simulink model "updated_target_driver_2026_withVariants_MPC"  (R2024b)
settings: Solver=FixedStepDiscrete  StartTime=0.0  StopTime=running_time  FixedStep=dt_s  RelTol=1e-3
values from neighbouring files (symbols this model uses):
  A = gamma_2*gamma_3*Thrust_desired    [force2voltage.m]
  a2_lb = -0.25    [target_driver_setup_2022_Ctrl_V_2_4.m]    (also in target_driver_setup_2022_Ctrl_V_2_4_geometric.m; target_driver_setup_mpc_12msdelay.m; target_driver_setup_mpc_andWLQP.m)
  a2_openloop = -0    (= 0)    [target_driver_setup_2022_Ctrl_V_2_4.m]    (also in target_driver_setup_2022_Ctrl_V_2_4_geometric.m; target_driver_setup_mpc_12msdelay.m; target_driver_setup_mpc_andWLQP.m)
  a2_ub = 0.25    [target_driver_setup_2022_Ctrl_V_2_4.m]    (also in target_driver_setup_2022_Ctrl_V_2_4_geometric.m; target_driver_setup_mpc_12msdelay.m; target_driver_setup_mpc_andWLQP.m)
  adaptive_flag = 0    [target_driver_setup_2022_Ctrl_V_2_4.m]    (also in target_driver_setup_2022_Ctrl_V_2_4_geometric.m; target_driver_setup_mpc_12msdelay.m = 1; target_driver_setup_mpc_andWLQP.m = 1)
  adaptive_gain = [gamma_adaptive, adaptive_roll_limit, adaptive_pitch_limit, adaptive_yaw_limit, c_2_adaptive, gamma_lateral_adaptive, adaptive_x_limit, adaptive_y_limit, adaptive_z_limit, c_1_adaptive]    [target_driver_setup_2022_Ctrl_V_2_4.m]    (also in target_driver_setup_2022_Ctrl_V_2_4_geometric.m; target_driver_setup_mpc_12msdelay.m; target_driver_setup_mpc_andWLQP.m)
  adaptive_lateral_flag = 0    [target_driver_setup_2022_Ctrl_V_2_4.m]    (also in target_driver_setup_2022_Ctrl_V_2_4_geometric.m; target_driver_setup_mpc_12msdelay.m = 1; target_driver_setup_mpc_andWLQP.m = 1)
  adaptive_pitch_init = 0    [target_driver_setup_2022_Ctrl_V_2_4.m]    (also in target_driver_setup_2022_Ctrl_V_2_4_geometric.m; target_driver_setup_mpc_12msdelay.m; target_driver_setup_mpc_andWLQP.m)
  adaptive_pitch_limit = 0.1/(scale^2)    (= 1e-07)    [target_driver_setup_2022_Ctrl_V_2_4.m]    (also in target_driver_setup_2022_Ctrl_V_2_4_geometric.m = 3e-07; target_driver_setup_mpc_12msdelay.m; target_driver_setup_mpc_andWLQP.m)
  adaptive_pitch_limit_low = -adaptive_pitch_limit    (= -1e-07)    [target_driver_setup_2022_Ctrl_V_2_4.m]    (also in target_driver_setup_2022_Ctrl_V_2_4_geometric.m = -3e-07; target_driver_setup_mpc_12msdelay.m; target_driver_setup_mpc_andWLQP.m)
  adaptive_roll_init = 0    [target_driver_setup_2022_Ctrl_V_2_4.m]    (also in target_driver_setup_2022_Ctrl_V_2_4_geometric.m; target_driver_setup_mpc_12msdelay.m; target_driver_setup_mpc_andWLQP.m)
  adaptive_roll_limit = 0.3/(scale^2)    (= 3e-07)    [target_driver_setup_2022_Ctrl_V_2_4.m]    (also in target_driver_setup_2022_Ctrl_V_2_4_geometric.m; target_driver_setup_mpc_12msdelay.m; target_driver_setup_mpc_andWLQP.m)
  adaptive_roll_limit_low = -adaptive_roll_limit    (= -3e-07)    [target_driver_setup_2022_Ctrl_V_2_4.m]    (also in target_driver_setup_2022_Ctrl_V_2_4_geometric.m; target_driver_setup_mpc_12msdelay.m; target_driver_setup_mpc_andWLQP.m)
  adaptive_x_init = 0    [target_driver_setup_2022_Ctrl_V_2_4.m]    (also in target_driver_setup_2022_Ctrl_V_2_4_geometric.m; target_driver_setup_mpc_12msdelay.m; target_driver_setup_mpc_andWLQP.m)
  adaptive_x_limit = 0.15/(scale)    (= 0.00015)    [target_driver_setup_2022_Ctrl_V_2_4.m]    (also in target_driver_setup_2022_Ctrl_V_2_4_geometric.m = 7.5e-05; target_driver_setup_mpc_12msdelay.m; target_driver_setup_mpc_andWLQP.m)
  adaptive_x_limit_low = -adaptive_x_limit    (= -0.00015)    [target_driver_setup_2022_Ctrl_V_2_4.m]    (also in target_driver_setup_2022_Ctrl_V_2_4_geometric.m = -7.5e-05; target_driver_setup_mpc_12msdelay.m; target_driver_setup_mpc_andWLQP.m)
  adaptive_y_init = 0    [target_driver_setup_2022_Ctrl_V_2_4.m]    (also in target_driver_setup_2022_Ctrl_V_2_4_geometric.m; target_driver_setup_mpc_12msdelay.m; target_driver_setup_mpc_andWLQP.m)
  adaptive_y_limit = 0.15/(scale)    (= 0.00015)    [target_driver_setup_2022_Ctrl_V_2_4.m]    (also in target_driver_setup_2022_Ctrl_V_2_4_geometric.m = 7.5e-05; target_driver_setup_mpc_12msdelay.m; target_driver_setup_mpc_andWLQP.m)
  adaptive_y_limit_low = -adaptive_y_limit    (= -0.00015)    [target_driver_setup_2022_Ctrl_V_2_4.m]    (also in target_driver_setup_2022_Ctrl_V_2_4_geometric.m = -7.5e-05; target_driver_setup_mpc_12msdelay.m; target_driver_setup_mpc_andWLQP.m)
  adaptive_yaw_init = 0    [target_driver_setup_2022_Ctrl_V_2_4.m]    (also in target_driver_setup_2022_Ctrl_V_2_4_geometric.m; target_driver_setup_mpc_12msdelay.m; target_driver_setup_mpc_andWLQP.m)
  adaptive_yaw_limit = 0.035/(scale^2)    (= 3.5e-08)    [target_driver_setup_2022_Ctrl_V_2_4.m]    (also in target_driver_setup_2022_Ctrl_V_2_4_geometric.m; target_driver_setup_mpc_12msdelay.m; target_driver_setup_mpc_andWLQP.m)
  adaptive_yaw_limit_low = -adaptive_yaw_limit    (= -3.5e-08)    [target_driver_setup_2022_Ctrl_V_2_4.m]    (also in target_driver_setup_2022_Ctrl_V_2_4_geometric.m; target_driver_setup_mpc_12msdelay.m; target_driver_setup_mpc_andWLQP.m)
  adaptive_z_init = 0/scale    (= 0)    [target_driver_setup_2022_Ctrl_V_2_4.m]    (also in target_driver_setup_2022_Ctrl_V_2_4_geometric.m; target_driver_setup_mpc_12msdelay.m; target_driver_setup_mpc_andWLQP.m)
  adaptive_z_limit = 0.20/(scale)    (= 0.0002)    [target_driver_setup_2022_Ctrl_V_2_4.m]    (also in target_driver_setup_2022_Ctrl_V_2_4_geometric.m = 0.0008; target_driver_setup_mpc_12msdelay.m = 0.0008; target_driver_setup_mpc_andWLQP.m = 0.0008)
  adaptive_z_limit_low = -adaptive_z_limit/1    (= -0.0002)    [target_driver_setup_2022_Ctrl_V_2_4.m]    (also in target_driver_setup_2022_Ctrl_V_2_4_geometric.m = -0.0008; target_driver_setup_mpc_12msdelay.m = -0.0008; target_driver_setup_mpc_andWLQP.m = -0.0008)
  att_s = 500    [target_driver_setup_2022_Ctrl_V_2_4.m]    (also in target_driver_setup_2022_Ctrl_V_2_4_geometric.m; target_driver_setup_mpc_12msdelay.m; target_driver_setup_mpc_andWLQP.m)
  b_1_d_desired = [1,0,0]    [target_driver_setup_2022_Ctrl_V_2_4.m]    (also in target_driver_setup_2022_Ctrl_V_2_4_geometric.m; target_driver_setup_mpc_12msdelay.m; target_driver_setup_mpc_andWLQP.m)
  closedloop_flag = 1    [target_driver_setup_2022_Ctrl_V_2_4.m]    (also in target_driver_setup_2022_Ctrl_V_2_4_geometric.m = 0; target_driver_setup_mpc_12msdelay.m = 0; target_driver_setup_mpc_andWLQP.m = 0)
  control_gain = [k_x,k_v, k_R, k_Omega, k_z, k_vz, k_Rx]    [target_driver_setup_2022_Ctrl_V_2_4.m]    (also in target_driver_setup_2022_Ctrl_V_2_4_geometric.m = [k_x,k_v,k_R,k_Omega_pitch,k_Omega_roll,k_z,k_vz,k_Rx]; target_driver_setup_mpc_12msdelay.m = [k_x, k_v, k_R, k_Omega, k_z, k_vz, k_Rx,                  k; target_driver_setup_mpc_andWLQP.m = [k_x, k_v, k_R, k_Omega, k_z, k_vz, k_Rx,                  k)
  delay = delay-vicon_sample_cycle/2    [target_driver_setup_2022_Ctrl_V_2_4.m]    (also in target_driver_setup_2022_Ctrl_V_2_4_geometric.m; target_driver_setup_mpc_12msdelay.m; target_driver_setup_mpc_andWLQP.m)
  drv_amp = abs((vleft_p2p-vright_p2p))/2+min(vleft_p2p,vright_p2p)    [Wing_traj_to_Voltage.m]    (also in force2voltage.m; target_driver_setup_2022_Ctrl_V_2_4.m = 300; target_driver_setup_2022_Ctrl_V_2_4_geometric.m = 133; target_driver_setup_mpc_12msdelay.m = 150)
  drv_bias = max_drv_bias    (= 300)    [target_driver_setup_2022_Ctrl_V_2_4.m]    (also in target_driver_setup_2022_Ctrl_V_2_4_geometric.m = 200; target_driver_setup_mpc_12msdelay.m = 200; target_driver_setup_mpc_andWLQP.m = 200)
  drv_pitch_left = vleft_pitch    [Wing_traj_to_Voltage.m]    (also in force2voltage.m = 0; target_driver_setup_2022_Ctrl_V_2_4.m = 0; target_driver_setup_2022_Ctrl_V_2_4_geometric.m = 0; target_driver_setup_mpc_12msdelay.m = 9.05)
  drv_pitch_right = vright_pitch    [Wing_traj_to_Voltage.m]    (also in force2voltage.m = 0; target_driver_setup_2022_Ctrl_V_2_4.m = 0; target_driver_setup_2022_Ctrl_V_2_4_geometric.m = 0; target_driver_setup_mpc_12msdelay.m = 9.05)
  drv_roll = (vleft_p2p-vright_p2p)/4    [Wing_traj_to_Voltage.m]    (also in force2voltage.m; target_driver_setup_2022_Ctrl_V_2_4.m = 0; target_driver_setup_2022_Ctrl_V_2_4_geometric.m = -0.001; target_driver_setup_mpc_12msdelay.m = -0.001)
  dt_s = 1e-3    (= 0.001)    [target_driver_setup_2022_Ctrl_V_2_4.m]    (also in target_driver_setup_2022_Ctrl_V_2_4_geometric.m = 0.0002; target_driver_setup_mpc_12msdelay.m = 0.0002; target_driver_setup_mpc_andWLQP.m = 0.0002)
  f_fin = f    (= 180)    [target_driver_setup_2022_Ctrl_V_2_4.m]    (also in target_driver_setup_2022_Ctrl_V_2_4_geometric.m = 155; target_driver_setup_mpc_12msdelay.m = 155; target_driver_setup_mpc_andWLQP.m = 155)
  f_int = f    (= 180)    [target_driver_setup_2022_Ctrl_V_2_4.m]    (also in target_driver_setup_2022_Ctrl_V_2_4_geometric.m = 155; target_driver_setup_mpc_12msdelay.m = 155; target_driver_setup_mpc_andWLQP.m = 155)
  g = 9.8    [target_driver_setup_2022_Ctrl_V_2_4.m]    (also in target_driver_setup_2022_Ctrl_V_2_4_geometric.m; target_driver_setup_mpc_12msdelay.m; target_driver_setup_mpc_andWLQP.m = 9.81; test_full_attitude_mpc.m = 9.81)
  I_moment_vec = [Ixx, Iyy, Izz]    [target_driver_setup_2022_Ctrl_V_2_4.m]    (also in target_driver_setup_2022_Ctrl_V_2_4_geometric.m; target_driver_setup_mpc_12msdelay.m; target_driver_setup_mpc_andWLQP.m)
  k_tau_vec = [k_tau_roll;k_tau_pitch]    [target_driver_setup_2022_Ctrl_V_2_4_geometric.m]    (also in target_driver_setup_mpc_12msdelay.m; target_driver_setup_mpc_andWLQP.m)
  landing_flag = 0    [target_driver_setup_2022_Ctrl_V_2_4.m]    (also in target_driver_setup_2022_Ctrl_V_2_4_geometric.m; target_driver_setup_mpc_12msdelay.m; target_driver_setup_mpc_andWLQP.m)
  landing_parameter = [start_delay+T,transition_rate, rising_time, falling_time, landing_rising_time, landing_z_decrease, landing_y_decrease, landing_x_decrease]    [target_driver_setup_2022_Ctrl_V_2_4.m]    (also in target_driver_setup_2022_Ctrl_V_2_4_geometric.m; target_driver_setup_mpc_12msdelay.m; target_driver_setup_mpc_andWLQP.m)
  low_bound = -8    [target_driver_setup_2022_Ctrl_V_2_4.m]    (also in target_driver_setup_2022_Ctrl_V_2_4_geometric.m = -5; target_driver_setup_mpc_12msdelay.m = -10; target_driver_setup_mpc_andWLQP.m = -10)
  low_bound_eR = -0.8    [target_driver_setup_2022_Ctrl_V_2_4.m]    (also in target_driver_setup_2022_Ctrl_V_2_4_geometric.m = -1.2; target_driver_setup_mpc_12msdelay.m = -1.2; target_driver_setup_mpc_andWLQP.m = -1.2)
  low_bound_vx = -0.5    [target_driver_setup_2022_Ctrl_V_2_4.m]    (also in target_driver_setup_2022_Ctrl_V_2_4_geometric.m; target_driver_setup_mpc_12msdelay.m; target_driver_setup_mpc_andWLQP.m)
  low_bound_vy = -0.5    [target_driver_setup_2022_Ctrl_V_2_4.m]    (also in target_driver_setup_2022_Ctrl_V_2_4_geometric.m; target_driver_setup_mpc_12msdelay.m; target_driver_setup_mpc_andWLQP.m)
  low_bound_vz = -0.5    [target_driver_setup_2022_Ctrl_V_2_4.m]    (also in target_driver_setup_2022_Ctrl_V_2_4_geometric.m; target_driver_setup_mpc_12msdelay.m; target_driver_setup_mpc_andWLQP.m)
  low_bound_x = -0.06    [target_driver_setup_2022_Ctrl_V_2_4.m]    (also in target_driver_setup_2022_Ctrl_V_2_4_geometric.m = -0.1; target_driver_setup_mpc_12msdelay.m = -0.6; target_driver_setup_mpc_andWLQP.m = -0.6)
  low_bound_y = -0.06    [target_driver_setup_2022_Ctrl_V_2_4.m]    (also in target_driver_setup_2022_Ctrl_V_2_4_geometric.m; target_driver_setup_mpc_12msdelay.m = -0.6; target_driver_setup_mpc_andWLQP.m = -0.6)
  low_bound_z = -0.04    [target_driver_setup_2022_Ctrl_V_2_4.m]    (also in target_driver_setup_2022_Ctrl_V_2_4_geometric.m; target_driver_setup_mpc_12msdelay.m = -0.1; target_driver_setup_mpc_andWLQP.m = -0.1)
  m = t <= t_zoom    [plot_roll_torque_cmd_vs_actual.m]    (also in plot_roll_torque_cmd_vs_actual_flightlog.m = t >= t0 & t <= t1; target_driver_setup_2022_Ctrl_V_2_4.m = 0.000124; target_driver_setup_2022_Ctrl_V_2_4_geometric.m = 8.5655e-05; target_driver_setup_mpc_12msdelay.m = 8.5655e-05)
  params_vec = [params_opt.delta_1, params_opt.delta_2, params_opt.delta_3,      params_opt.gamma_1, params_opt.gamma_2_1, params_opt.gamma_3,      params_opt.eta, params_opt.nu, params_opt.mu]'    [force2voltage_tuningSandbox.m]    (also in target_driver_setup_2022_Ctrl_V_2_4.m = [params_opt.delta_1, params_opt.delta_2, params_opt.delta_3,; target_driver_setup_2022_Ctrl_V_2_4_geometric.m = [params_opt.delta_1, params_opt.delta_2, params_opt.delta_3,; target_driver_setup_mpc_12msdelay.m = [params_opt.delta_1, params_opt.delta_2, params_opt.delta_3,; target_driver_setup_mpc_andWLQP.m = [params_opt.delta_1, params_opt.delta_2, params_opt.delta_3,)
  phase = 0    [target_driver_setup_2022_Ctrl_V_2_4.m]    (also in target_driver_setup_2022_Ctrl_V_2_4_geometric.m; target_driver_setup_mpc_12msdelay.m; target_driver_setup_mpc_andWLQP.m)
  r_desired = [default_x, default_y,z_desired]    [target_driver_setup_2022_Ctrl_V_2_4.m]    (also in target_driver_setup_2022_Ctrl_V_2_4_geometric.m; target_driver_setup_mpc_12msdelay.m; target_driver_setup_mpc_andWLQP.m)
  roll_offset_angle = 0    [target_driver_setup_2022_Ctrl_V_2_4.m]    (also in target_driver_setup_2022_Ctrl_V_2_4_geometric.m; target_driver_setup_mpc_12msdelay.m; target_driver_setup_mpc_andWLQP.m)
  running_time = start_delay+total_T    (= 9)    [target_driver_setup_2022_Ctrl_V_2_4.m]    (also in target_driver_setup_2022_Ctrl_V_2_4_geometric.m = 10; target_driver_setup_mpc_12msdelay.m = 0.5; target_driver_setup_mpc_andWLQP.m = 10)
  running_time_control = start_delay_control+total_T+0.0    (= 7.1)    [target_driver_setup_2022_Ctrl_V_2_4.m]    (also in target_driver_setup_2022_Ctrl_V_2_4_geometric.m = 10; target_driver_setup_mpc_12msdelay.m = 0.5; target_driver_setup_mpc_andWLQP.m = 10)
  sampling_f = 10000    [target_driver_setup_2022_Ctrl_V_2_4.m]    (also in target_driver_setup_2022_Ctrl_V_2_4_geometric.m = 5000; target_driver_setup_mpc_12msdelay.m = 5000; target_driver_setup_mpc_andWLQP.m = 5000)
  start_delay = 2.0    (= 2)    [target_driver_setup_2022_Ctrl_V_2_4.m]    (also in target_driver_setup_2022_Ctrl_V_2_4_geometric.m = 0; target_driver_setup_mpc_12msdelay.m = 0; target_driver_setup_mpc_andWLQP.m = 0)
  start_delay_control = start_delay + ramp_delay    (= 0.1)    [target_driver_setup_2022_Ctrl_V_2_4.m]    (also in target_driver_setup_2022_Ctrl_V_2_4_geometric.m = 0; target_driver_setup_mpc_12msdelay.m = 0; target_driver_setup_mpc_andWLQP.m = 0)
  T = 1    [target_driver_setup_2022_Ctrl_V_2_4.m]    (also in target_driver_setup_2022_Ctrl_V_2_4_geometric.m = 10; target_driver_setup_mpc_12msdelay.m = 0.5; target_driver_setup_mpc_andWLQP.m = 10; test_full_attitude_mpc.m = T0 + nu(1))
  task_flag = 0    [target_driver_setup_2022_Ctrl_V_2_4.m]    (also in target_driver_setup_2022_Ctrl_V_2_4_geometric.m; target_driver_setup_mpc_12msdelay.m; target_driver_setup_mpc_andWLQP.m)
  task_parameter = [radius_ref, frequency_ref, radius_ratio, lissajous_ratio, lissajous_delta, lissajous_amplitude_ratio,z_radius_ratio]    [target_driver_setup_2022_Ctrl_V_2_4.m]    (also in target_driver_setup_2022_Ctrl_V_2_4_geometric.m; target_driver_setup_mpc_12msdelay.m; target_driver_setup_mpc_andWLQP.m)
  upp_bound = 8    [target_driver_setup_2022_Ctrl_V_2_4.m]    (also in target_driver_setup_2022_Ctrl_V_2_4_geometric.m = 5; target_driver_setup_mpc_12msdelay.m = 10; target_driver_setup_mpc_andWLQP.m = 10)
  upp_bound_eR = 0.8    [target_driver_setup_2022_Ctrl_V_2_4.m]    (also in target_driver_setup_2022_Ctrl_V_2_4_geometric.m = 1.2; target_driver_setup_mpc_12msdelay.m = 1.2; target_driver_setup_mpc_andWLQP.m = 1.2)
  upp_bound_vx = 0.5    [target_driver_setup_2022_Ctrl_V_2_4.m]    (also in target_driver_setup_2022_Ctrl_V_2_4_geometric.m; target_driver_setup_mpc_12msdelay.m; target_driver_setup_mpc_andWLQP.m)
  upp_bound_vy = 0.5    [target_driver_setup_2022_Ctrl_V_2_4.m]    (also in target_driver_setup_2022_Ctrl_V_2_4_geometric.m; target_driver_setup_mpc_12msdelay.m; target_driver_setup_mpc_andWLQP.m)
  upp_bound_vz = 0.5    [target_driver_setup_2022_Ctrl_V_2_4.m]    (also in target_driver_setup_2022_Ctrl_V_2_4_geometric.m; target_driver_setup_mpc_12msdelay.m; target_driver_setup_mpc_andWLQP.m)
  upp_bound_x = 0.06    [target_driver_setup_2022_Ctrl_V_2_4.m]    (also in target_driver_setup_2022_Ctrl_V_2_4_geometric.m = 0.1; target_driver_setup_mpc_12msdelay.m = 0.6; target_driver_setup_mpc_andWLQP.m = 0.6)
  upp_bound_y = 0.06    [target_driver_setup_2022_Ctrl_V_2_4.m]    (also in target_driver_setup_2022_Ctrl_V_2_4_geometric.m; target_driver_setup_mpc_12msdelay.m = 0.6; target_driver_setup_mpc_andWLQP.m = 0.6)
  upp_bound_z = 0.04    [target_driver_setup_2022_Ctrl_V_2_4.m]    (also in target_driver_setup_2022_Ctrl_V_2_4_geometric.m; target_driver_setup_mpc_12msdelay.m = 0.1; target_driver_setup_mpc_andWLQP.m = 0.1)
  weights_vec = [ws; wds; wpr_xy;wpr_z; wpf; wvr_xy; wvr_z ... (first row only)    [target_driver_setup_2022_Ctrl_V_2_4_geometric.m]    (also in target_driver_setup_mpc_12msdelay.m; target_driver_setup_mpc_andWLQP.m)
undefined symbols (not defined in the file or in its folder): Com1, DiscIntNeverNeededParam, dspblkCoreblockFVToolHelper, gcbh, left_mapping, left_mapping_F_to_Phi, lp_den, lp_num, none, right_mapping, right_mapping_F_to_Phi, vlp_den, vlp_num
libraries: simulink x20, xpcseriallib x2, cstblocks x1, xpcnilib x1, xpcutilitieslib x1
(part 5 of 7)

== matlab function updated_target_driver_2026_withVariants_MPC/Geometric Controller/lateral adaptive/Adaptive Control ==
  data: current_adaptive_x input; current_adaptive_y input; current_adaptive_z input; der_adaptive_torque_x output size=[1 1]; e_x input; e_v input; adaptive_gain_limit input; der_adaptive_torque_y output size=[1 1]; der_adaptive_torque_z output size=[1 1]
function [der_adaptive_torque_x, der_adaptive_torque_y, der_adaptive_torque_z] = fcn(current_adaptive_x,current_adaptive_y,current_adaptive_z, e_x,e_v,adaptive_gain_limit)


% Current state of adaptation
adaptive_torque_x=current_adaptive_x;
adaptive_torque_y=current_adaptive_y;
adaptive_torque_z=current_adaptive_z;

% Adaptive control parameters
gamma_lateral_adaptive = adaptive_gain_limit(6);
adaptvie_x_limit = adaptive_gain_limit(7);
adaptvie_y_limit = adaptive_gain_limit(8);
adaptvie_z_limit = adaptive_gain_limit(9);
c_1 = adaptive_gain_limit(10);

% Flag indicating the limit
adaptive_flag_x = adaptive_torque_x*(e_v(1)+c_1*e_x(1));
adaptive_flag_y = adaptive_torque_y*(e_v(2)+c_1*e_x(2));
adaptive_flag_z = adaptive_torque_z*(e_v(3)+c_1*e_x(3));

% size(adaptive_flag_x)

% derivative for desired adaptation
der_adaptive = gamma_lateral_adaptive*(e_v+c_1*e_x);

% epsillon=1e-15;


if (adaptive_flag_x<=0 && abs(adaptive_torque_x)==adaptvie_x_limit) || abs(adaptive_torque_x)<adaptvie_x_limit
	
	der_adaptive_torque_x=der_adaptive(1);
else
	der_adaptive_torque_x = 0;
end

if (adaptive_flag_y<=0 && abs(adaptive_torque_y)==adaptvie_y_limit) || abs(adaptive_torque_y)<adaptvie_y_limit
	
	der_adaptive_torque_y=der_adaptive(2);
else
	der_adaptive_torque_y = 0;
	
end

if (adaptive_flag_z<=0 && abs(adaptive_torque_z)==adaptvie_z_limit)|| abs(adaptive_torque_z)<adaptvie_z_limit
	
	der_adaptive_torque_z=der_adaptive(3);
else
	der_adaptive_torque_z = 0;
	
end


end

== matlab function updated_target_driver_2026_withVariants_MPC/Variant Subsystem/Simulation/Drake 2 Controller Axes1 ==
  data: x_drake input; x output; y_drake input; z_drake input; y output; z output
function [x,y,z] = fcn(x_drake,y_drake,z_drake)

    [x,y,z] = drake2controllerposition(x_drake,y_drake,z_drake); 

end

== matlab function updated_target_driver_2026_withVariants_MPC/Desired attitude and normalized error/Variant Subsystem/saturated normalized error observation/Saturated angular velocity eOmega /Compute attitude error eR ==
  data: y output size=[3 1]; R_cur input; R_desired input; omega input; omega_desired input
function y  = fcn(R_cur,R_desired,omega, omega_desired)

Rot_cur = [R_cur(1), R_cur(2), R_cur(3); R_cur(4), R_cur(5), R_cur(6); R_cur(7), R_cur(8), R_cur(9)];
Rot_desired = [R_desired(1), R_desired(2), R_desired(3); R_desired(4), R_desired(5), R_desired(6); R_desired(7), R_desired(8), R_desired(9)];
eOmega=zeros(3,1);
eOmega = omega - Rot_cur'*Rot_desired*omega_desired;

y = eOmega;

end

== matlab function updated_target_driver_2026_withVariants_MPC/Desired attitude and normalized error/Variant Subsystem/saturated normalized error observation/Saturated normalized eR/Compute attitude error eR ==
  data: y output size=[3 1]; R_cur input; R_desired input
function y  = fcn(R_cur,R_desired)

Rot_cur = [R_cur(1), R_cur(2), R_cur(3); R_cur(4), R_cur(5), R_cur(6); R_cur(7), R_cur(8), R_cur(9)];
Rot_desired = [R_desired(1), R_desired(2), R_desired(3); R_desired(4), R_desired(5), R_desired(6); R_desired(7), R_desired(8), R_desired(9)];
eR_so3=zeros(3,3);
eR_so3 = 1/2*(Rot_desired.'*Rot_cur-Rot_cur.'*Rot_desired);

eR = zeros(3,1);
eR(1) = eR_so3(3,2);
eR(2) = eR_so3(1,3);
eR(3) = eR_so3(2,1);

y = eR;

% Rot_desired 
end

== matlab function updated_target_driver_2026_withVariants_MPC/Force to voltage/Control Mode/Force_to_Voltage1/Desired_Force_to_Voltage ==
  data: Thrust_desired input; drv_amp output; Roll_torque_desired input; Pitch_torque_desired input; Yaw_torque_desired input; drv_roll output; drv_pitch_left output; drv_pitch_right output; a2_coeff output; params_vec input
function [drv_amp, drv_roll, drv_pitch_left, drv_pitch_right, a2_coeff] =    fcn(Thrust_desired, Roll_torque_desired, Pitch_torque_desired, Yaw_torque_desired, params_vec)

% 
% Thrust_desired = 0.7e-3;% N
% Roll_torque_desired = 20e-6; %mN mm 
% Pitch_torque_desired = 0;% N  
% Yaw_torque_desired = 0;  
[drv_amp, drv_roll, drv_pitch_left, drv_pitch_right, a2_coeff] = force2voltage( ...
    Thrust_desired, Roll_torque_desired, Pitch_torque_desired, ...
    Yaw_torque_desired, params_vec);
% % global params_opt
% 
% delta_1 = params_vec(1);
% delta_2 = params_vec(2);
% delta_3 = params_vec(3);
% gamma_1 = params_vec(4);
% gamma_2 = params_vec(5);
% gamma_3 = params_vec(6);
% eta = params_vec(7);
% nu = params_vec(8);
% mu = params_vec(9);
% 
% 
% % Initializing for averaging filter at the end to prevent InF
% if Thrust_desired==0    
%     u4 = 0;
% else
%     u4 = Pitch_torque_desired/(Thrust_desired*delta_3*gamma_2)-nu;
% end
% 
% 
% % u3 calculation when tau approaches to zero
% if abs(Yaw_torque_desired)<1e-12
% 
%    u3 = -mu;
% else
%     % Bounds for the mapping to produce real solution
%     lb =(Thrust_desired/2)*(gamma_2*gamma_3*delta_2*mu/delta_1-sqrt((gamma_2*gamma_3*delta_2*Thrust_desired*mu/delta_1)^2+gamma_2*gamma_3));
%     ub =(Thrust_desired/2)*(gamma_2*gamma_3*delta_2*mu/delta_1+sqrt((gamma_2*gamma_3*delta_2*Thrust_desired*mu/delta_1)^2+gamma_2*gamma_3));
% 
%     if Yaw_torque_desired>=ub
%        Yaw_torque_desired = ub;
%     elseif Yaw_torque_desired<=lb
%        Yaw_torque_desired = lb; 
%     end
% 
%     % u3 calculation when tau approaches zero
%     if abs(Yaw_torque_desired) < 1e-12
%         u3 = -mu;
%     else
%         A = gamma_2*gamma_3*Thrust_desired;
%         B = gamma_2*gamma_3*delta_2*Thrust_desired*mu/delta_1;
% 
%         disc = A^2 - 4*Yaw_torque_desired*(Yaw_torque_desired - B);
% 
%     % Numerical / feasibility guard
%     if disc < 0
%         disc = 0;
%     end
% 
%     u3 = delta_1*(A - sqrt(disc))/(2*delta_2*Yaw_torque_desired);
%     end
% end
% 
% D = delta_1^2+delta_2^2*u3^2;
% % gamma_2*Thrust_desired+Roll_torque_desired 
% u1 = (gamma_2*Thrust_desired+Roll_torque_desired)/(2*gamma_1*gamma_2*D*eta);
% u2 = (gamma_2*Thrust_desired-Roll_torque_desired)/(2*gamma_1*gamma_2*D);
% 
% u1 = max(u1, 0); 
% u2 = max(u2, 0); % Guard against negative voltage
% vleft_p2p = sqrt(u1)*2; 
% vright_p2p = sqrt(u2)*2;
% vleft_pitch = u4;
% vright_pitch = u4;
% 
% 
% drv_amp = abs((vleft_p2p-vright_p2p))/2+min(vleft_p2p,vright_p2p); % p2p
% drv_roll = (vleft_p2p-vright_p2p)/4; % Amplitude
% drv_pitch_left = vleft_pitch;
% drv_pitch_right = vright_pitch;
% a2_coeff = u3;
% 
end

== matlab function updated_target_driver_2026_withVariants_MPC/Desired attitude and normalized error/Variant Subsystem/unsaturated normalized error observation1/Saturated angular velocity eOmega /Compute attitude error eR ==
  data: y output size=[3 1]; R_cur input; R_desired input; omega input; omega_desired input
function y  = fcn(R_cur,R_desired,omega, omega_desired)

Rot_cur = [R_cur(1), R_cur(2), R_cur(3); R_cur(4), R_cur(5), R_cur(6); R_cur(7), R_cur(8), R_cur(9)];
Rot_desired = [R_desired(1), R_desired(2), R_desired(3); R_desired(4), R_desired(5), R_desired(6); R_desired(7), R_desired(8), R_desired(9)];
eOmega=zeros(3,1);
eOmega = omega - Rot_cur'*Rot_desired*omega_desired;

y = eOmega;

end

== matlab function updated_target_driver_2026_withVariants_MPC/Desired attitude and normalized error/Variant Subsystem/unsaturated normalized error observation1/Saturated normalized eR/Compute attitude error eR ==
  data: y output size=[3 1]; R_cur input; R_desired input
function y  = fcn(R_cur,R_desired)

Rot_cur = [R_cur(1), R_cur(2), R_cur(3); R_cur(4), R_cur(5), R_cur(6); R_cur(7), R_cur(8), R_cur(9)];
Rot_desired = [R_desired(1), R_desired(2), R_desired(3); R_desired(4), R_desired(5), R_desired(6); R_desired(7), R_desired(8), R_desired(9)];
eR_so3=zeros(3,3);
eR_so3 = 1/2*(Rot_desired.'*Rot_cur-Rot_cur.'*Rot_desired);

eR = zeros(3,1);
eR(1) = eR_so3(3,2);
eR(2) = eR_so3(1,3);
eR(3) = eR_so3(2,1);

y = eR;

% Rot_desired 
end

== matlab function updated_target_driver_2026_withVariants_MPC/Force to voltage/Control Mode/Force_to_Voltage1/Force to Trajectory  ==
  data: Thrust_desired input; Phi_left_p2p_desired output; Roll_torque_desired input; Pitch_torque_desired input; left_mapping_F_to_Phi input; right_mapping_F_to_Phi input; A input; Phi_right_p2p_desired output; Phi_pitch_desired output
function [Phi_left_p2p_desired, Phi_right_p2p_desired, Phi_pitch_desired] = fcn(Thrust_desired, Roll_torque_desired, Pitch_torque_desired, left_mapping_F_to_Phi, right_mapping_F_to_Phi, A)

delta_opt_L = left_mapping_F_to_Phi(1);
gamma_opt_L = left_mapping_F_to_Phi(2);
phi_opt_L = left_mapping_F_to_Phi(3);
phi_opt_offset_L = left_mapping_F_to_Phi(4);

delta_opt_R = right_mapping_F_to_Phi(1);
gamma_opt_R = right_mapping_F_to_Phi(2);
phi_opt_R = right_mapping_F_to_Phi(3);
phi_opt_offset_R = right_mapping_F_to_Phi(4);

T_thrust_roll = A*[ delta_opt_L              ,               delta_opt_R;...
                    delta_opt_L*gamma_opt_L  , - delta_opt_R*gamma_opt_R];
T_pitch_thrust = A*[delta_opt_L*gamma_opt_L  , delta_opt_R*gamma_opt_R].*[phi_opt_L, phi_opt_R];
T_pitch_offset = A*[delta_opt_L*gamma_opt_L  , delta_opt_R*gamma_opt_R].*[phi_opt_offset_L, phi_opt_offset_R];

Thrust_roll = [Thrust_desired; Roll_torque_desired];
u1_u2_desired = (T_thrust_roll)\Thrust_roll;

if (T_pitch_thrust*u1_u2_desired)==0
	Phi_pitch_desired = 0;
else
	Phi_pitch_desired = (Pitch_torque_desired-T_pitch_offset*u1_u2_desired)/(T_pitch_thrust*u1_u2_desired);
end

Phi_left_p2p_desired = sqrt(u1_u2_desired(1));
Phi_right_p2p_desired = sqrt(u1_u2_desired(2));

== matlab function updated_target_driver_2026_withVariants_MPC/Force to voltage/Control Mode/Force_to_Voltage1/Trajectory to Voltage Input  ==
  data: Phi_left_p2p_command input; drv_amp output; Phi_right_p2p_command input; Phi_pitch_command input; drv_roll output; drv_pitch_left output; left_mapping input; right_mapping input; drv_pitch_right output
function [drv_amp, drv_roll, drv_pitch_left, drv_pitch_right] = fcn(Phi_left_p2p_command,Phi_right_p2p_command,Phi_pitch_command,left_mapping,right_mapping)

% Mapping for Voltage peak to peak from desired Stroke peak to peak
p1_left = left_mapping(1); % V_left_p2p = p1_left*Phi_p2p + p2_left
p2_left = left_mapping(2);
p1_right = right_mapping(1); % V_right_p2p = p1_right*Phi_p2p + p2_right
p2_right = right_mapping(2);

% Mapping for Voltage offset to peak from desired Stroke peak to peak
p1_pitch_left = left_mapping(3); % vleft_pitch = p1_pitch_left*Phi_pitch_command + p2_pitch_left
p2_pitch_left = left_mapping(4);
p1_pitch_right = right_mapping(3); % vright_pitch = p1_pitch_right*Phi_pitch_command + p2_pitch_right
p2_pitch_right = right_mapping(4);

vleft_p2p = p1_left*Phi_left_p2p_command + p2_left;
vright_p2p = p1_right*Phi_right_p2p_command + p2_right;
vleft_pitch = p1_pitch_left*Phi_pitch_command + p2_pitch_left;
vright_pitch = p1_pitch_right*Phi_pitch_command + p2_pitch_right;



drv_amp = abs((vleft_p2p-vright_p2p))/2+min(vleft_p2p,vright_p2p); % p2p
drv_roll = (vleft_p2p-vright_p2p)/4; % Amplitude
drv_pitch_left = vleft_pitch;
drv_pitch_right = vright_pitch;

== matlab function updated_target_driver_2026_withVariants_MPC/Force to voltage/Replay Mode/Force_to_Voltage1/Desired_Force_to_Voltage ==
  data: Thrust_desired input; drv_amp output; Roll_torque_desired input; Pitch_torque_desired input; Yaw_torque_desired input; drv_roll output; drv_pitch_left output; drv_pitch_right output; a2_coeff output; params_vec input
function [drv_amp, drv_roll, drv_pitch_left, drv_pitch_right, a2_coeff] =    fcn(Thrust_desired, Roll_torque_desired, Pitch_torque_desired, Yaw_torque_desired, params_vec)

% 
% Thrust_desired = 0.7e-3;% N
% Roll_torque_desired = 20e-6; %mN mm 
% Pitch_torque_desired = 0;% N  
% Yaw_torque_desired = 0;  
[drv_amp, drv_roll, drv_pitch_left, drv_pitch_right, a2_coeff] = force2voltage( ...
    Thrust_desired, Roll_torque_desired, Pitch_torque_desired, ...
    Yaw_torque_desired, params_vec);
% % global params_opt
% 
% delta_1 = params_vec(1);
% delta_2 = params_vec(2);
% delta_3 = params_vec(3);
% gamma_1 = params_vec(4);
% gamma_2 = params_vec(5);
% gamma_3 = params_vec(6);
% eta = params_vec(7);
% nu = params_vec(8);
% mu = params_vec(9);
% 
% 
% % Initializing for averaging filter at the end to prevent InF
% if Thrust_desired==0    
%     u4 = 0;
% else
%     u4 = Pitch_torque_desired/(Thrust_desired*delta_3*gamma_2)-nu;
% end
% 
% 
% % u3 calculation when tau approaches to zero
% if abs(Yaw_torque_desired)<1e-12
% 
%    u3 = -mu;
% else
%     % Bounds for the mapping to produce real solution
%     lb =(Thrust_desired/2)*(gamma_2*gamma_3*delta_2*mu/delta_1-sqrt((gamma_2*gamma_3*delta_2*Thrust_desired*mu/delta_1)^2+gamma_2*gamma_3));
%     ub =(Thrust_desired/2)*(gamma_2*gamma_3*delta_2*mu/delta_1+sqrt((gamma_2*gamma_3*delta_2*Thrust_desired*mu/delta_1)^2+gamma_2*gamma_3));
% 
%     if Yaw_torque_desired>=ub
%        Yaw_torque_desired = ub;
%     elseif Yaw_torque_desired<=lb
%        Yaw_torque_desired = lb; 
%     end
% 
%     % u3 calculation when tau approaches zero
%     if abs(Yaw_torque_desired) < 1e-12
%         u3 = -mu;
%     else
%         A = gamma_2*gamma_3*Thrust_desired;
%         B = gamma_2*gamma_3*delta_2*Thrust_desired*mu/delta_1;
% 
%         disc = A^2 - 4*Yaw_torque_desired*(Yaw_torque_desired - B);
% 
%     % Numerical / feasibility guard
%     if disc < 0
%         disc = 0;
%     end
% 
%     u3 = delta_1*(A - sqrt(disc))/(2*delta_2*Yaw_torque_desired);
%     end
% end
% 
% D = delta_1^2+delta_2^2*u3^2;
% % gamma_2*Thrust_desired+Roll_torque_desired 
% u1 = (gamma_2*Thrust_desired+Roll_torque_desired)/(2*gamma_1*gamma_2*D*eta);
% u2 = (gamma_2*Thrust_desired-Roll_torque_desired)/(2*gamma_1*gamma_2*D);
% 
% u1 = max(u1, 0); 
% u2 = max(u2, 0); % Guard against negative voltage
% vleft_p2p = sqrt(u1)*2; 
% vright_p2p = sqrt(u2)*2;
% vleft_pitch = u4;
% vright_pitch = u4;
% 
% 
% drv_amp = abs((vleft_p2p-vright_p2p))/2+min(vleft_p2p,vright_p2p); % p2p
% drv_roll = (vleft_p2p-vright_p2p)/4; % Amplitude
% drv_pitch_left = vleft_pitch;
% drv_pitch_right = vright_pitch;
% a2_coeff = u3;
% 
end

== matlab function updated_target_driver_2026_withVariants_MPC/Force to voltage/Replay Mode/Force_to_Voltage1/Force to Trajectory  ==
  data: Thrust_desired input; Phi_left_p2p_desired output; Roll_torque_desired input; Pitch_torque_desired input; left_mapping_F_to_Phi input; right_mapping_F_to_Phi input; A input; Phi_right_p2p_desired output; Phi_pitch_desired output
function [Phi_left_p2p_desired, Phi_right_p2p_desired, Phi_pitch_desired] = fcn(Thrust_desired, Roll_torque_desired, Pitch_torque_desired, left_mapping_F_to_Phi, right_mapping_F_to_Phi, A)

delta_opt_L = left_mapping_F_to_Phi(1);
gamma_opt_L = left_mapping_F_to_Phi(2);
phi_opt_L = left_mapping_F_to_Phi(3);
phi_opt_offset_L = left_mapping_F_to_Phi(4);

delta_opt_R = right_mapping_F_to_Phi(1);
gamma_opt_R = right_mapping_F_to_Phi(2);
phi_opt_R = right_mapping_F_to_Phi(3);
phi_opt_offset_R = right_mapping_F_to_Phi(4);

T_thrust_roll = A*[ delta_opt_L              ,               delta_opt_R;...
                    delta_opt_L*gamma_opt_L  , - delta_opt_R*gamma_opt_R];
T_pitch_thrust = A*[delta_opt_L*gamma_opt_L  , delta_opt_R*gamma_opt_R].*[phi_opt_L, phi_opt_R];
T_pitch_offset = A*[delta_opt_L*gamma_opt_L  , delta_opt_R*gamma_opt_R].*[phi_opt_offset_L, phi_opt_offset_R];

Thrust_roll = [Thrust_desired; Roll_torque_desired];
u1_u2_desired = (T_thrust_roll)\Thrust_roll;

if (T_pitch_thrust*u1_u2_desired)==0
	Phi_pitch_desired = 0;
else
	Phi_pitch_desired = (Pitch_torque_desired-T_pitch_offset*u1_u2_desired)/(T_pitch_thrust*u1_u2_desired);
end

Phi_left_p2p_desired = sqrt(u1_u2_desired(1));
Phi_right_p2p_desired = sqrt(u1_u2_desired(2));

== matlab function updated_target_driver_2026_withVariants_MPC/Desired attitude and normalized error/Desired_Attitude  ==
  data: R_cur input; R_d_prev input; R_d_vec output; e_x input; e_v input; x_d_ddot input; b_1_d input; control_gain input; m input; g input; update input; adaptive_lateral_control input
function R_d_vec = fcn(R_cur,R_d_prev, e_x,e_v,x_d_ddot, b_1_d, control_gain, m, g, update, adaptive_lateral_control)
%#codegen
% FEEDBACK-FREE attitude reference for the monolithic upright MPC.
%
% The old geometric version tilted R_desired with -K_X.*e_x - K_V.*e_v
% (a position controller). The MPC in the controller block now owns ALL
% position feedback, so the desired body-z here is pure feed-forward:
% gravity compensation plus desired acceleration from the trajectory.
% For hover this makes R_desired level (b_3_d = e_3) with the commanded
% heading. Inputs e_x, e_v, control_gain, adaptive_lateral_control are
% kept for signature compatibility but unused.
R_d_vec = zeros(9,1);
if update>0
   R_d_vec=R_d_prev;
else
    e_3 = [0 0 1]';
    b_1_d = b_1_d/norm(b_1_d);
    f_ff = m*g*e_3 + m*reshape(x_d_ddot,3,1);
    b_3_d = f_ff / max(norm(f_ff), 1e-12);
    b_2_d = cross(b_3_d,b_1_d) / max(norm(cross(b_3_d,b_1_d)), 1e-12);
    R_d = [cross(b_2_d,b_3_d) b_2_d b_3_d];
    R_d_vec = [R_d(1,1); R_d(1,2); R_d(1,3); R_d(2,1); R_d(2,2); R_d(2,3); R_d(3,1); R_d(3,2); R_d(3,3)];
end
end

== matlab function updated_target_driver_2026_withVariants_MPC/Force to voltage/Replay Mode/Force_to_Voltage1/Trajectory to Voltage Input  ==
  data: Phi_left_p2p_command input; drv_amp output; Phi_right_p2p_command input; Phi_pitch_command input; drv_roll output; drv_pitch_left output; left_mapping input; right_mapping input; drv_pitch_right output
function [drv_amp, drv_roll, drv_pitch_left, drv_pitch_right] = fcn(Phi_left_p2p_command,Phi_right_p2p_command,Phi_pitch_command,left_mapping,right_mapping)

% Mapping for Voltage peak to peak from desired Stroke peak to peak
p1_left = left_mapping(1); % V_left_p2p = p1_left*Phi_p2p + p2_left
p2_left = left_mapping(2);
p1_right = right_mapping(1); % V_right_p2p = p1_right*Phi_p2p + p2_right
p2_right = right_mapping(2);

% Mapping for Voltage offset to peak from desired Stroke peak to peak
p1_pitch_left = left_mapping(3); % vleft_pitch = p1_pitch_left*Phi_pitch_command + p2_pitch_left
p2_pitch_left = left_mapping(4);
p1_pitch_right = right_mapping(3); % vright_pitch = p1_pitch_right*Phi_pitch_command + p2_pitch_right
p2_pitch_right = right_mapping(4);

vleft_p2p = p1_left*Phi_left_p2p_command + p2_left;
vright_p2p = p1_right*Phi_right_p2p_command + p2_right;
vleft_pitch = p1_pitch_left*Phi_pitch_command + p2_pitch_left;
vright_pitch = p1_pitch_right*Phi_pitch_command + p2_pitch_right;



drv_amp = abs((vleft_p2p-vright_p2p))/2+min(vleft_p2p,vright_p2p); % p2p
drv_roll = (vleft_p2p-vright_p2p)/4; % Amplitude
drv_pitch_left = vleft_pitch;
drv_pitch_right = vright_pitch;

== matlab function updated_target_driver_2026_withVariants_MPC/Desired attitude and normalized error/Geometric derivative for Rd in SO(3)/First order geometric derivative in SO(3)  ==
  data: R_prev input; omega_d output size=[3 1]; R_cur input; omega_d_prev input; update input; count input; sampling_f input
function omega_d   = fcn(R_prev, R_cur, omega_d_prev, update, count, sampling_f)

Rot_cur = [R_cur(1), R_cur(2), R_cur(3); R_cur(4), R_cur(5), R_cur(6); R_cur(7), R_cur(8), R_cur(9)];
Rot_prev = [R_prev(1), R_prev(2), R_prev(3); R_prev(4), R_prev(5), R_prev(6); R_prev(7), R_prev(8), R_prev(9)];

R_diff = Rot_prev'*Rot_cur;

tr_R_diff = trace(R_diff);
omega_d = zeros(3,1);
% omega_d_dot = zeros(3,1);

if update>0
   omega_d=omega_d_prev; 
%    omega_d_dot = omega_d_dot_prev;
else
    
% isreal(tr_R_diff)
if abs((tr_R_diff-1)/2)<=1
    theta = acos((tr_R_diff-1)/2);
else
    theta=acos((tr_R_diff-1)/2/abs((tr_R_diff-1)/2));
end

if theta==0
	theta=1e-14;
end

   w = 1/(2*sin(theta))*[R_diff(3,2)-R_diff(2,3); R_diff(1,3) - R_diff(3,1); R_diff(2,1)-R_diff(1,2)];
   % omega_d = w*theta*10000/(count+1);
   omega_d = w*theta*sampling_f/(count+1);
%    omega_d_dot = (omega_d - omega_d_prev)*10000/(count+1);
     
end
% 
% if theta==0 %update~=0 
%     y = y_prev;
% else
%      w = 1/(2*sin(theta))*[R_diff(3,2)-R_diff(2,3); R_diff(1,3) - R_diff(3,1); R_diff(2,1)-R_diff(1,2)];
%      y = w*theta*10000/20;
% end

== matlab function updated_target_driver_2026_withVariants_MPC/Force_to_Voltage1/Desired_Force_to_Voltage ==
  data: Thrust_desired input; drv_amp output; Roll_torque_desired input; Pitch_torque_desired input; Yaw_torque_desired input; drv_roll output; drv_pitch_left output; drv_pitch_right output; a2_coeff output; params_vec input
function [drv_amp, drv_roll, drv_pitch_left, drv_pitch_right, a2_coeff] =    fcn(Thrust_desired, Roll_torque_desired, Pitch_torque_desired, Yaw_torque_desired, params_vec)

% 
% Thrust_desired = 0.7e-3;% N
% Roll_torque_desired = 20e-6; %mN mm 
% Pitch_torque_desired = 0;% N  
% Yaw_torque_desired = 0;  
[drv_amp, drv_roll, drv_pitch_left, drv_pitch_right, a2_coeff] = force2voltage( ...
    Thrust_desired, Roll_torque_desired, Pitch_torque_desired, ...
    Yaw_torque_desired, params_vec);
% % global params_opt
% 
% delta_1 = params_vec(1);
% delta_2 = params_vec(2);
% delta_3 = params_vec(3);
% gamma_1 = params_vec(4);
% gamma_2 = params_vec(5);
% gamma_3 = params_vec(6);
% eta = params_vec(7);
% nu = params_vec(8);
% mu = params_vec(9);
% 
% 
% % Initializing for averaging filter at the end to prevent InF
% if Thrust_desired==0    
%     u4 = 0;
% else
%     u4 = Pitch_torque_desired/(Thrust_desired*delta_3*gamma_2)-nu;
% end
% 
% 
% % u3 calculation when tau approaches to zero
% if abs(Yaw_torque_desired)<1e-12
% 
%    u3 = -mu;
% else
%     % Bounds for the mapping to produce real solution
%     lb =(Thrust_desired/2)*(gamma_2*gamma_3*delta_2*mu/delta_1-sqrt((gamma_2*gamma_3*delta_2*Thrust_desired*mu/delta_1)^2+gamma_2*gamma_3));
%     ub =(Thrust_desired/2)*(gamma_2*gamma_3*delta_2*mu/delta_1+sqrt((gamma_2*gamma_3*delta_2*Thrust_desired*mu/delta_1)^2+gamma_2*gamma_3));
% 
%     if Yaw_torque_desired>=ub
%        Yaw_torque_desired = ub;
%     elseif Yaw_torque_desired<=lb
%        Yaw_torque_desired = lb; 
%     end
% 
%     % u3 calculation when tau approaches zero
%     if abs(Yaw_torque_desired) < 1e-12
%         u3 = -mu;
%     else
%         A = gamma_2*gamma_3*Thrust_desired;
%         B = gamma_2*gamma_3*delta_2*Thrust_desired*mu/delta_1;
% 
%         disc = A^2 - 4*Yaw_torque_desired*(Yaw_torque_desired - B);
% 
%     % Numerical / feasibility guard
%     if disc < 0
%         disc = 0;
%     end
% 
%     u3 = delta_1*(A - sqrt(disc))/(2*delta_2*Yaw_torque_desired);
%     end
% end
% 
% D = delta_1^2+delta_2^2*u3^2;
% % gamma_2*Thrust_desired+Roll_torque_desired 
% u1 = (gamma_2*Thrust_desired+Roll_torque_desired)/(2*gamma_1*gamma_2*D*eta);
% u2 = (gamma_2*Thrust_desired-Roll_torque_desired)/(2*gamma_1*gamma_2*D);
% 
% u1 = max(u1, 0); 
% u2 = max(u2, 0); % Guard against negative voltage
% vleft_p2p = sqrt(u1)*2; 
% vright_p2p = sqrt(u2)*2;
% vleft_pitch = u4;
% vright_pitch = u4;
% 
% 
% drv_amp = abs((vleft_p2p-vright_p2p))/2+min(vleft_p2p,vright_p2p); % p2p
% drv_roll = (vleft_p2p-vright_p2p)/4; % Amplitude
% drv_pitch_left = vleft_pitch;
% drv_pitch_right = vright_pitch;
% a2_coeff = u3;
% 
end

== matlab function updated_target_driver_2026_withVariants_MPC/Geometric Controller/Attitude Adaptive/Adaptive Control ==
  data: current_adaptive_roll input; current_adaptive_pitch input; current_adaptive_yaw input; der_adaptive_torque_roll output size=[1 1]; e_R input; e_Omega input; adaptive_gain_limit input; der_adaptive_torque_pitch output size=[1 1]; der_adaptive_torque_yaw output size=[1 1]
function [der_adaptive_torque_roll, der_adaptive_torque_pitch, der_adaptive_torque_yaw] = fcn(current_adaptive_roll,current_adaptive_pitch,current_adaptive_yaw, e_R,e_Omega,adaptive_gain_limit)


% Current state of adaptation
adaptive_torque_roll=current_adaptive_roll;
adaptive_torque_pitch=current_adaptive_pitch;
adaptive_torque_yaw=current_adaptive_yaw;

% Adaptive control parameters
gamma_adaptive = adaptive_gain_limit(1);
adaptvie_roll_limit = adaptive_gain_limit(2);
adaptvie_pitch_limit = adaptive_gain_limit(3);
adaptvie_yaw_limit = adaptive_gain_limit(4);
c_2 = adaptive_gain_limit(5);

% Flag indicating the limit
adaptive_flag_roll = adaptive_torque_roll*(e_Omega(1)+c_2*e_R(1));
adaptive_flag_pitch = adaptive_torque_pitch*(e_Omega(2)+c_2*e_R(2));
adaptive_flag_yaw = adaptive_torque_yaw*(e_Omega(3)+c_2*e_R(3));

% size(adaptive_flag_roll)

% derivative for desired adaptation
der_adaptive = gamma_adaptive*(e_Omega+c_2*e_R);

% epsillon=1e-15;


if (adaptive_flag_roll<=0 && abs(adaptive_torque_roll)==adaptvie_roll_limit) || abs(adaptive_torque_roll)<adaptvie_roll_limit
	
	der_adaptive_torque_roll=der_adaptive(1);
else
	der_adaptive_torque_roll = 0;
end

if (adaptive_flag_pitch<=0 && abs(adaptive_torque_pitch)==adaptvie_pitch_limit) || abs(adaptive_torque_pitch)<adaptvie_pitch_limit
	
	der_adaptive_torque_pitch=der_adaptive(2);
else
	der_adaptive_torque_pitch = 0;
	
end

if (adaptive_flag_yaw<=0 && abs(adaptive_torque_yaw)==adaptvie_yaw_limit)|| abs(adaptive_torque_yaw)<adaptvie_yaw_limit
	
	der_adaptive_torque_yaw=der_adaptive(3);
else
	der_adaptive_torque_yaw = 0;
	
end


end

== matlab function updated_target_driver_2026_withVariants_MPC/Variant Subsystem/Simulation/Drake 2 Controller Axes ==
  data: alpha input; rol_c output; beta input; gamma input; pitch_c output; yaw_c output
function [rol_c,pitch_c,yaw_c] = fcn(alpha,beta,gamma)

    [rol_c,pitch_c,yaw_c] = drake2controller(alpha,beta,gamma); 

end

== matlab function updated_target_driver_2026_withVariants_MPC/Force_to_Voltage1/Force to Trajectory  ==
  data: Thrust_desired input; Phi_left_p2p_desired output; Roll_torque_desired input; Pitch_torque_desired input; left_mapping_F_to_Phi input; right_mapping_F_to_Phi input; A input; Phi_right_p2p_desired output; Phi_pitch_desired output
function [Phi_left_p2p_desired, Phi_right_p2p_desired, Phi_pitch_desired] = fcn(Thrust_desired, Roll_torque_desired, Pitch_torque_desired, left_mapping_F_to_Phi, right_mapping_F_to_Phi, A)

delta_opt_L = left_mapping_F_to_Phi(1);
gamma_opt_L = left_mapping_F_to_Phi(2);
phi_opt_L = left_mapping_F_to_Phi(3);
phi_opt_offset_L = left_mapping_F_to_Phi(4);

delta_opt_R = right_mapping_F_to_Phi(1);
gamma_opt_R = right_mapping_F_to_Phi(2);
phi_opt_R = right_mapping_F_to_Phi(3);
phi_opt_offset_R = right_mapping_F_to_Phi(4);

T_thrust_roll = A*[ delta_opt_L              ,               delta_opt_R;...
                    delta_opt_L*gamma_opt_L  , - delta_opt_R*gamma_opt_R];
T_pitch_thrust = A*[delta_opt_L*gamma_opt_L  , delta_opt_R*gamma_opt_R].*[phi_opt_L, phi_opt_R];
T_pitch_offset = A*[delta_opt_L*gamma_opt_L  , delta_opt_R*gamma_opt_R].*[phi_opt_offset_L, phi_opt_offset_R];

Thrust_roll = [Thrust_desired; Roll_torque_desired];
u1_u2_desired = (T_thrust_roll)\Thrust_roll;

if (T_pitch_thrust*u1_u2_desired)==0
	Phi_pitch_desired = 0;
else
	Phi_pitch_desired = (Pitch_torque_desired-T_pitch_offset*u1_u2_desired)/(T_pitch_thrust*u1_u2_desired);
end

Phi_left_p2p_desired = sqrt(u1_u2_desired(1));
Phi_right_p2p_desired = sqrt(u1_u2_desired(2));
